simulink model "Controll_RigidBody_R2021b"  (R2021b)
settings: Solver=ode4  StartTime=0.0  StopTime=inf  FixedStep=0.01  MaxStep=0.2  RelTol=1e-3
values from neighbouring files (symbols this model uses):
  Km1 = Km_gain    (= 0.1)    [param_EiH_VFC.m]
  Km2 = Km_gain    (= 0.1)    [param_EiH_VFC.m]
  Km3 = Km_gain    (= 0.1)    [param_EiH_VFC.m]
  Km4 = Km_gain    (= 0.1)    [param_EiH_VFC.m]
  Km5 = Km_gain    (= 0.1)    [param_EiH_VFC.m]
  Km6 = Km_gain    (= 0.1)    [param_EiH_VFC.m]
  R_threshold = 1e-8    (= 1e-08)    [param_EiH_VFC.m]
  zeta_threshold = 1e-8    (= 1e-08)    [param_EiH_VFC.m]
undefined symbols (not defined in the file or in its folder): magnitude, pzeta_d
libraries: dspnetwork x2, dspmtrx3 x1
(part 1 of 2)
settings Model: Creator=toshiyuki  LastModifiedBy=takeh
settings SolverCC: AlgebraicLoopSolver=TrustRegion  InsertRTBMode=Always
settings DataIOCC: ReturnWorkspaceOutputs=off  ReturnWorkspaceOutputsName=tp4a89a2fa_3ce3_4014_a3ba_d599f69fb3ba
settings DebuggingCC: SFMachineParentedDataDiag=warning  ArithmeticOperatorsInVariantConditions=warning
settings SFSimCC: SimUseLocalCustomCode=off  CustomCodeUndefinedFunction=UseInterfaceOnly
settings RTWCC: RTWUseLocalCustomCode=off

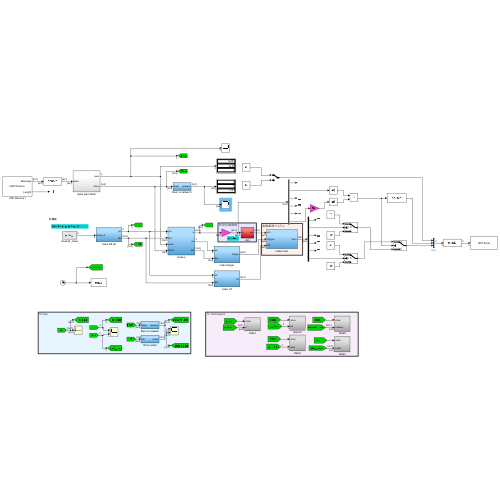
[thumbnail: Simulink's stored preview of the top-level diagram]
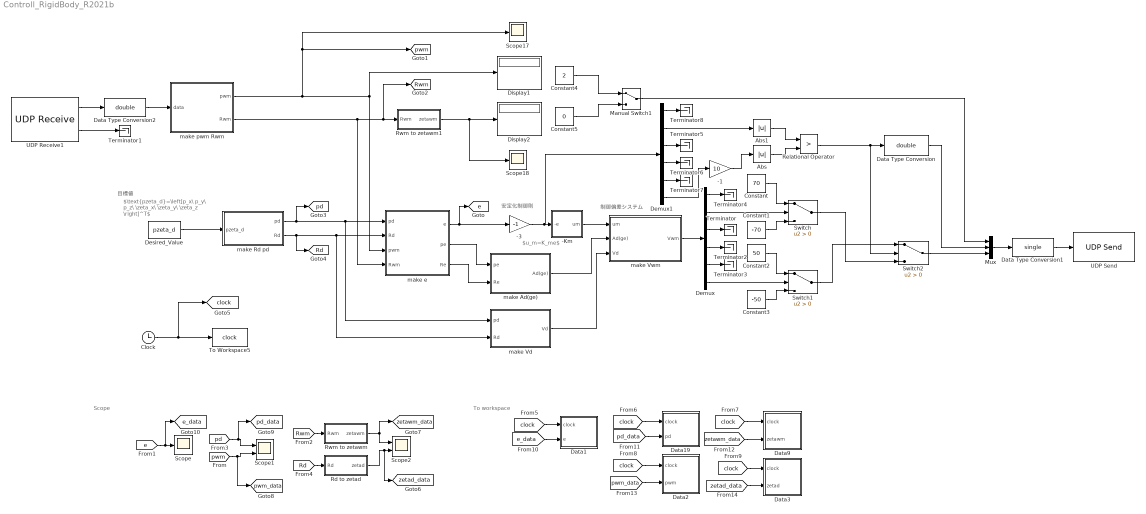
== system Controll_RigidBody_R2021b ==
  note: 制御偏差システム
  note: 目標値
  note: 安定化制御則
  note: $\text{pzeta_d}=\left[p_x\ p_y\ p_z\ \zeta_x\ \zeta_y\ \zeta_z \right]^T$
  note: Scope
  note: To workspace
  note: $u_m=K_me$
  -1 : Gain  Gain=10  SaturateOnIntegerOverflow=on  OutDataTypeStr=Inherit: Same as input  ParamDataTypeStr=Inherit: Same as input
  -3 : Gain  Gain=-1  SaturateOnIntegerOverflow=on  OutDataTypeStr=Inherit: Same as input  ParamDataTypeStr=Inherit: Same as input
  -Km : Subsystem
  Abs : Abs
  Abs1 : Abs
  Clock : Clock
  Constant : Constant  Value=70
  Constant1 : Constant  Value=-70
  Constant2 : Constant  Value=50
  Constant3 : Constant  Value=-50
  Constant4 : Constant  Value=2
  Constant5 : Constant  Value=0
  Data Type Conversion : DataTypeConversion  OutDataTypeStr=double
  Data Type Conversion1 : DataTypeConversion  OutDataTypeStr=single
  Data Type Conversion2 : DataTypeConversion  OutDataTypeStr=double
  Data1 : Subsystem
  Data19 : Subsystem
  Data2 : Subsystem
  Data3 : Subsystem
  Data9 : Subsystem
  Demux : Demux  Outputs=6
  Demux1 : Demux  Outputs=6
  Desired_Value : Constant  Value=pzeta_d
  Display1 : Display
  Display2 : Display
  Manual Switch1 : ManualSwitch
  Mux : Mux  Inputs=3
  Rd to zetad : Subsystem
  Relational Operator : RelationalOperator  Operator=>  OutDataTypeStr=boolean  RndMeth=Simplest
  Rwm to zetawm : Subsystem
  Rwm to zetawm1 : Subsystem
  Scope : Scope
  Scope1 : Scope  NumInputPorts=2
  Scope17 : Scope
  Scope18 : Scope
  Scope2 : Scope  NumInputPorts=2
  Switch : Switch  Criteria=u2 > Threshold
  Switch1 : Switch  Criteria=u2 > Threshold
  Switch2 : Switch  Criteria=u2 > Threshold
  Terminator{,1..8} (9 alike) : Terminator
  To Workspace5 : ToWorkspace  VariableName=clock  SaveFormat=Structure  SampleTime=-1
  UDP Receive1 : dspnetwork/UDP Receive  localURL='0.0.0.0'  localPort=51000  remoteURL='127.0.0.1'  remotePort=-1  recvBufferSize=24  dims=6  signalDatatype=single  isComplex=off  isVarSize=off  showBlockingTime=off  blockingTime=0  sampletime=-1  blockPlatform=[]
  UDP Send : dspnetwork/UDP Send  remoteURL='127.0.0.1'  remotePort=52000  localURL='0.0.0.0'  localPortSource=Automatically determine  localPort=-1  sendBufferSize=8192  sampletime=-1  blockPlatform=[]  separateLengthPort=0
  make Ad(ge) : Subsystem
  make Rd pd : Subsystem
  make Vd : Subsystem
  make Vwm : Subsystem
  make e : Subsystem
  make pwm Rwm : Subsystem
  tag scope: Rd=global, Rwm=global, clock=global, e=global, e_data=global, pd=global, pd_data=global, pwm=global, pwm_data=global, zetad_data=global, zetawm_data=global
  wires:
  make Rd pd/1(pd) -> [pd], make e/1(pd), make Vd/1(pd)
  make Rd pd/2(Rd) -> [Rd], make e/2(Rd), make Vd/2(Rd)
  Desired_Value/1 -> make Rd pd/1(pzeta_d)
  make e/1(e) -> [e], -3/1
  make e/2(pe) -> make Ad(ge)/1(pe)
  make e/3(Re) -> make Ad(ge)/2(Re)
  -Km/1(um) -> make Vwm/1(um)
  make Ad(ge)/1(Ad(ge)) -> make Vwm/2(Ad(ge))
  make Vd/1(Vd) -> make Vwm/3(Vd)
  make Vwm/1(Vwm) -> Demux/1
  make pwm Rwm/2(Rwm) -> [Rwm], Rwm to zetawm1/1(Rwm), make e/4(Rwm)
  make pwm Rwm/1(pwm) -> [pwm], Scope17/1, make e/3(pwm), Display1/1
  [e] -> [e_data], Scope/1
  [pd] -> [pd_data], Scope1/1
  [pwm] -> [pwm_data], Scope1/2
  [Rwm] -> Rwm to zetawm/1(Rwm)
  [Rd] -> Rd to zetad/1(Rd)
  Rwm to zetawm/1(zetawm) -> [zetawm_data], Scope2/1
  Rd to zetad/1(zetad) -> [zetad_data], Scope2/2
  Clock/1 -> [clock], To Workspace5/1
  [clock] -> Data1/1(clock)
  [clock] -> Data19/1(clock)
  [clock] -> Data9/1(clock)
  [clock] -> Data2/1(clock)
  [clock] -> Data3/1(clock)
  [zetawm_data] -> Data9/2(zetawm)
  [zetad_data] -> Data3/2(zetad)
  [pd_data] -> Data19/2(pd)
  [pwm_data] -> Data2/2(pwm)
  [e_data] -> Data1/2(e)
  UDP Receive1/1 -> Data Type Conversion2/1
  UDP Receive1/2 -> Terminator1/1
  Data Type Conversion2/1 -> make pwm Rwm/1(data)
  Rwm to zetawm1/1(zetawm) -> Scope18/1, Display2/1
  Demux/3 -> Terminator/1
  Demux/4 -> Terminator2/1
  Demux/5 -> Terminator3/1
  Demux/1 -> Terminator4/1
  Demux/2 -> Switch/2
  Constant/1 -> Switch/1
  Constant1/1 -> Switch/3
  Demux/6 -> Switch1/2
  Constant2/1 -> Switch1/1
  Constant3/1 -> Switch1/3
  Data Type Conversion1/1 -> UDP Send/1
  Mux/1 -> Data Type Conversion1/1
  Constant4/1 -> Manual Switch1/1
  Constant5/1 -> Manual Switch1/2
  Demux1/4 -> Terminator6/1
  Demux1/5 -> Terminator7/1
  Demux1/1 -> Terminator8/1
  Demux1/2 -> Abs1/1
  Demux1/3 -> Terminator5/1
  Demux1/6 -> -1/1
  -3/1 -> Demux1/1, -Km/1(-e)
  -1/1 -> Abs/1
  Abs1/1 -> Relational Operator/1
  Abs/1 -> Relational Operator/2
  Relational Operator/1 -> Switch2/2, Data Type Conversion/1
  Manual Switch1/1 -> Mux/1
  Switch/1 -> Switch2/3
  Switch2/1 -> Mux/3
  Switch1/1 -> Switch2/1
  Data Type Conversion/1 -> Mux/2

== system Controll_RigidBody_R2021b/-Km ==
  -e : Inport
  Gain : Gain  Gain=-1  Multiplication=Matrix(K*u)  SaturateOnIntegerOverflow=on  OutDataTypeStr=Inherit: Same as input  ParamDataTypeStr=Inherit: Same as input
  Kcc : Subsystem
  Product : Product  Multiplication=Matrix(*)  InputSameDT=on  SaturateOnIntegerOverflow=on  OutDataTypeStr=Inherit: Same as first input
  um : Outport  VectorParamsAs1DForOutWhenUnconnected=off
  wires:
  Gain/1 -> Product/1
  Kcc/1(Km) -> Gain/1
  Product/1 -> um/1
  -e/1 -> Product/2

== system Controll_RigidBody_R2021b/Data1 ==
  clock : Inport
  e : Inport  Port=2
  Demux4 : Demux  Outputs=6
      settings: DisplayOption=none
  Mux2 : Mux  Inputs=7
  To Workspace1 : ToWorkspace  VariableName=e  SaveFormat=Structure  SampleTime=-1
  wires:
  Demux4/6 -> Mux2/7
  Demux4/5 -> Mux2/6
  Demux4/4 -> Mux2/5
  Demux4/3 -> Mux2/4
  Demux4/2 -> Mux2/3
  Demux4/1 -> Mux2/2
  clock/1 -> Mux2/1
  Mux2/1 -> To Workspace1/1
  e/1 -> Demux4/1

== system Controll_RigidBody_R2021b/Data19 ==
  clock : Inport
  pd : Inport  Port=2
  Demux4 : Demux  Outputs=3
      settings: DisplayOption=none
  Mux2 : Mux
  To Workspace1 : ToWorkspace  VariableName=pd  SaveFormat=Structure  SampleTime=-1
  wires:
  pd/1 -> Demux4/1
  clock/1 -> Mux2/1
  Mux2/1 -> To Workspace1/1
  Demux4/3 -> Mux2/4
  Demux4/2 -> Mux2/3
  Demux4/1 -> Mux2/2

== system Controll_RigidBody_R2021b/Data2 ==
  clock : Inport
  pwm : Inport  Port=2
  Demux4 : Demux  Outputs=3
      settings: DisplayOption=none
  Mux2 : Mux
  To Workspace1 : ToWorkspace  VariableName=pwm  SaveFormat=Structure  SampleTime=-1
  wires:
  Demux4/1 -> Mux2/2
  Demux4/2 -> Mux2/3
  Demux4/3 -> Mux2/4
  Mux2/1 -> To Workspace1/1
  clock/1 -> Mux2/1
  pwm/1 -> Demux4/1

== system Controll_RigidBody_R2021b/Data3 ==
  clock : Inport
  zetad : Inport  Port=2
  Demux4 : Demux  Outputs=3
      settings: DisplayOption=none
  Mux2 : Mux
  To Workspace1 : ToWorkspace  VariableName=zetad  SaveFormat=Structure  SampleTime=-1
  wires:
  zetad/1 -> Demux4/1
  clock/1 -> Mux2/1
  Mux2/1 -> To Workspace1/1
  Demux4/3 -> Mux2/4
  Demux4/2 -> Mux2/3
  Demux4/1 -> Mux2/2

== system Controll_RigidBody_R2021b/Data9 ==
  clock : Inport
  zetawm : Inport  Port=2
  Demux4 : Demux  Outputs=3
      settings: DisplayOption=none
  Mux2 : Mux
  To Workspace1 : ToWorkspace  VariableName=zetawm  SaveFormat=Structure  SampleTime=-1
  wires:
  Demux4/1 -> Mux2/2
  Demux4/2 -> Mux2/3
  Demux4/3 -> Mux2/4
  Mux2/1 -> To Workspace1/1
  clock/1 -> Mux2/1
  zetawm/1 -> Demux4/1

== system Controll_RigidBody_R2021b/Rd to zetad ==
  Rd : Inport
  e_R(R) : Subsystem
  make zeta : Subsystem
  zetad : Outport  VectorParamsAs1DForOutWhenUnconnected=off
  wires:
  make zeta/1(zeta) -> zetad/1
  Rd/1 -> e_R(R)/1(R)
  e_R(R)/1(sk(R)^vee) -> make zeta/1(sk(R)^vee)

== system Controll_RigidBody_R2021b/Rwm to zetawm ==
  Rwm : Inport
  e_R(R) : Subsystem
  make zeta : Subsystem
  zetawm : Outport  VectorParamsAs1DForOutWhenUnconnected=off
  wires:
  make zeta/1(zeta) -> zetawm/1
  Rwm/1 -> e_R(R)/1(R)
  e_R(R)/1(sk(R)^vee) -> make zeta/1(sk(R)^vee)

== system Controll_RigidBody_R2021b/Rwm to zetawm1 ==
  Rwm : Inport
  e_R(R) : Subsystem
  make zeta : Subsystem
  zetawm : Outport  VectorParamsAs1DForOutWhenUnconnected=off
  wires:
  make zeta/1(zeta) -> zetawm/1
  Rwm/1 -> e_R(R)/1(R)
  e_R(R)/1(sk(R)^vee) -> make zeta/1(sk(R)^vee)

== system Controll_RigidBody_R2021b/make Ad(ge) ==
  note: $\hat{p_e}R_e$
  note: $\left(R_e\ \hat{p_e}R_e\right)$
  note: $\left(0\ R_e\right)$
  note: $\text{Ad}_{(g_e)}=\left[\begin{array}{cc} R_e & \hat{p_e}R_e\\ 0&R_e \end{array}\right]$
  pe : Inport
  Re : Inport  Port=2
  Gain : Gain  Gain=0  Multiplication=Matrix(K*u)
  Identity Matrix : dspmtrx3/Identity Matrix  Inherit=off  N=3  Ts=1  dataType=double  isSigned=on  wordLen=16  udDataType=sfix(16)  fracBitsMode=Best precision  numFracBits=15  OutDataTypeStr=double  LastOutDataTypeStr=double
  Matrix Concatenate : Concatenate  Mode=Multidimensional array  ConcatenateDimension=2
  Matrix Concatenate1 : Concatenate  Mode=Multidimensional array  ConcatenateDimension=2
  Matrix Concatenate2 : Concatenate  Mode=Multidimensional array
  Product2 : Product  Multiplication=Matrix(*)
  wedge : Subsystem
  Ad(ge) : Outport  VectorParamsAs1DForOutWhenUnconnected=off
  wires:
  pe/1 -> wedge/1("[3x1]")
  wedge/1("[3x3]") -> Product2/1
  Re/1 -> Matrix Concatenate1/2, Product2/2, Matrix Concatenate/1
  Product2/1 -> Matrix Concatenate/2
  Matrix Concatenate/1 -> Matrix Concatenate2/1
  Matrix Concatenate1/1 -> Matrix Concatenate2/2
  Matrix Concatenate2/1 -> Ad(ge)/1
  Identity Matrix/1 -> Gain/1
  Gain/1 -> Matrix Concatenate1/1

== system Controll_RigidBody_R2021b/make Rd pd ==
  note: 目標姿勢
  note: 目標位置
  note: $p_d=\left(p_x \ p_y\ p_z\right)^T$$
  note: $\zeta_d=\left(\zeta_x \ \zeta_y\ \zeta_z\right)^T\text{\ \ →\ \ 回転行列}R_d$
  pzeta_d : Inport
  Demux3 : Demux  Outputs=6
      settings: DisplayOption=none
  Mux : Mux  Inputs=3
  Mux1 : Mux  Inputs=3
  make_Rd : Subsystem
  pd : Outport  VectorParamsAs1DForOutWhenUnconnected=off
  Rd : Outport  Port=2  VectorParamsAs1DForOutWhenUnconnected=off
  wires:
  Demux3/2 -> Mux1/2
  Demux3/1 -> Mux1/1
  Demux3/5 -> Mux/2
  Demux3/4 -> Mux/1
  pzeta_d/1 -> Demux3/1
  Mux/1 -> make_Rd/1(zeta_d)
  Demux3/3 -> Mux1/3
  Demux3/6 -> Mux/3
  Mux1/1 -> pd/1
  make_Rd/1(Rd) -> Rd/1

== system Controll_RigidBody_R2021b/make Vd ==
  note: $v_d^b=R_{d}^T\dot{p}_{d}$
  note: $\omega_d^b=\left(R_{d}^T\dot{R}_{d}\right)^\vee$
  note: $V_d^b=\left[\begin{array}{c} v_d^b\\ \omega_d^b \end{array} \right]$
  pd : Inport
  Rd : Inport  Port=2
  Derivative : Derivative
  Derivative1 : Derivative
  Math Function : Math  Operator=transpose  SignedPower=on  SaturateOnIntegerOverflow=on
  Mux : Mux  Inputs=2
  Product1 : Product  Multiplication=Matrix(*)
  Product2 : Product  Multiplication=Matrix(*)
  vee : Subsystem
  Vd : Outport  VectorParamsAs1DForOutWhenUnconnected=off
  wires:
  pd/1 -> Derivative/1
  Rd/1 -> Derivative1/1, Math Function/1
  Math Function/1 -> Product2/1, Product1/1
  Derivative1/1 -> Product1/2
  Product1/1 -> vee/1("[3*3]")
  vee/1("[3*1]") -> Mux/2
  Product2/1 -> Mux/1
  Mux/1 -> Vd/1
  Derivative/1 -> Product2/2

== system Controll_RigidBody_R2021b/make Vwm ==
  note: $\text{Ad}_{(g_e)}\ \ \text{→}\ \ \text{Ad}_{(g_e)}^{-1}$
  note: $V_{wm}=-\text{Ad}_{(g_e)}^{-1}\left(u_m-V_d\right)$
  um : Inport
  Ad(ge) : Inport  Port=2
  Vd : Inport  Port=3
  -3 : Gain  Gain=-1  SaturateOnIntegerOverflow=on  OutDataTypeStr=Inherit: Same as input  ParamDataTypeStr=Inherit: Same as input
  MATLAB Function : MATLAB Function  TreatAsAtomicUnit=on
  Product2 : Product  Multiplication=Matrix(*)
  Sum : Sum  Inputs=|+-
  Vwm : Outport  VectorParamsAs1DForOutWhenUnconnected=off
  wires:
  Product2/1 -> Vwm/1
  Ad(ge)/1 -> MATLAB Function/1(Ad_ge)
  um/1 -> Sum/1
  Vd/1 -> Sum/2
  MATLAB Function/1(inv_Ad_ge) -> -3/1
  -3/1 -> Product2/1
  Sum/1 -> Product2/2

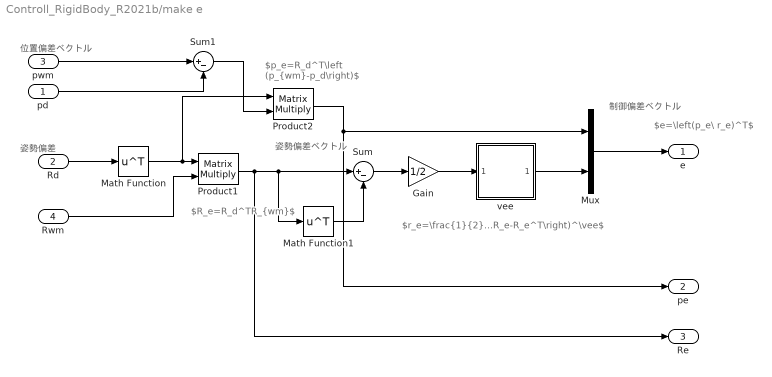
== system Controll_RigidBody_R2021b/make e ==
  note: 制御偏差ベクトル
  note: 姿勢偏差ベクトル
  note: 姿勢偏差
  note: 位置偏差ベクトル
  note: $p_e=R_d^T\left (p_{wm}-p_d\right)$
  note: $R_e=R_d^TR_{wm}$
  note: $r_e=\frac{1}{2}\left(R_e-R_e^T\right)^\vee$
  note: $e=\left(p_e\ r_e)^T$
  pd : Inport
  Rd : Inport  Port=2
  pwm : Inport  Port=3
  Rwm : Inport  Port=4
  Gain : Gain  Gain=1/2
  Math Function : Math  Operator=transpose  SignedPower=on  SaturateOnIntegerOverflow=on
  Math Function1 : Math  Operator=transpose  SignedPower=on  SaturateOnIntegerOverflow=on
  Mux : Mux  Inputs=2
  Product1 : Product  Multiplication=Matrix(*)
  Product2 : Product  Multiplication=Matrix(*)
  Sum : Sum  Inputs=|+-
  Sum1 : Sum  Inputs=|+-
  vee : Subsystem
  e : Outport  VectorParamsAs1DForOutWhenUnconnected=off
  pe : Outport  Port=2  VectorParamsAs1DForOutWhenUnconnected=off
  Re : Outport  Port=3  VectorParamsAs1DForOutWhenUnconnected=off
  wires:
  Rd/1 -> Math Function/1
  Math Function/1 -> Product2/1, Product1/1
  Rwm/1 -> Product1/2
  pwm/1 -> Sum1/1
  pd/1 -> Sum1/2
  Sum1/1 -> Product2/2
  vee/1("[3*1]") -> Mux/2
  Sum/1 -> Gain/1
  Math Function1/1 -> Sum/2
  Product2/1 -> pe/1, Mux/1
  Gain/1 -> vee/1("[3*3]")
  Mux/1 -> e/1
  Product1/1 -> Re/1, Math Function1/1, Sum/1

== system Controll_RigidBody_R2021b/make pwm Rwm ==
  data : Inport
  Constant : Constant  Value=0
  Demux : Demux  Outputs=6
  Mux1 : Mux  Inputs=3
  Mux2 : Mux  Inputs=3
  Sum5 : Sum  Inputs=|+-
  Sum6 : Sum  Inputs=|+-
  Sum7 : Sum  Inputs=+-|
  make_Rd : Subsystem
  pwm : Outport
  Rwm : Outport  Port=2
  wires:
  Sum6/1 -> Mux1/2
  Demux/6 -> Sum7/2
  Demux/4 -> Sum5/2
  Sum5/1 -> Mux1/1
  Demux/3 -> Sum7/1
  Demux/2 -> Sum6/1
  Demux/1 -> Sum5/1
  Demux/5 -> Sum6/2
  data/1 -> Demux/1
  Constant/1 -> Mux2/2, Mux2/1, Mux1/3
  Mux1/1 -> pwm/1
  Sum7/1 -> Mux2/3
  Mux2/1 -> make_Rd/1(zeta_d)
  make_Rd/1(Rd) -> Rwm/1

== system Controll_RigidBody_R2021b/-Km/Kcc ==
  Ke1 : Constant  Value=Km1
  Ke2 : Constant  Value=Km2
  Ke3 : Constant  Value=Km3
  Ke4 : Constant  Value=Km4
  Ke5 : Constant  Value=Km5
  Ke6 : Constant  Value=Km6
  Mux : Mux  Inputs=6
  diag : Subsystem
  Km : Outport  VectorParamsAs1DForOutWhenUnconnected=off
  wires:
  Mux/1 -> diag/1(in[6*1])
  Ke6/1 -> Mux/6
  Ke5/1 -> Mux/5
  Ke4/1 -> Mux/4
  Ke3/1 -> Mux/3
  Ke2/1 -> Mux/2
  Ke1/1 -> Mux/1
  diag/1(diag) -> Km/1

== system Controll_RigidBody_R2021b/Rd to zetad/e_R(R) ==
  R : Inport
  sk(R) : Subsystem
  vee : Subsystem
  sk(R)^vee : Outport  VectorParamsAs1DForOutWhenUnconnected=off
  wires:
  R/1 -> sk(R)/1(R)
  vee/1("[3*1]") -> sk(R)^vee/1
  sk(R)/1(sk(R)) -> vee/1("[3*3]")

== system Controll_RigidBody_R2021b/Rd to zetad/make zeta ==
  sk(R)^vee : Inport
  "3x1 -> 2norm" : Subsystem
  Product : Product  InputSameDT=on  SaturateOnIntegerOverflow=on  OutDataTypeStr=Inherit: Same as first input
  Product1 : Product  Inputs=/  InputSameDT=on  SaturateOnIntegerOverflow=on  OutDataTypeStr=Inherit: Same as first input
  Product2 : Product  InputSameDT=on  SaturateOnIntegerOverflow=on  OutDataTypeStr=Inherit: Same as first input
  Switch : Switch  Threshold=zeta_threshold  SaturateOnIntegerOverflow=on  InputSameDT=on
  Trigonometric Function : Trigonometry  Operator=asin
  zero : Constant  Value=[0;0;0]  VectorParams1D=off
  zero check zeta_threshold : Subsystem
  zeta : Outport  VectorParamsAs1DForOutWhenUnconnected=off
  wires:
  zero/1 -> Switch/3
  Product/1 -> Switch/1
  Switch/1 -> zeta/1
  zero check zeta_threshold/1(Out1) -> Switch/2, Product1/1, Trigonometric Function/1
  sk(R)^vee/1 -> "3x1 -> 2norm"/1(3x1), Product/2
  "3x1 -> 2norm"/1(2 norm) -> zero check zeta_threshold/1(In1)
  Trigonometric Function/1 -> Product2/1
  Product1/1 -> Product2/2
  Product2/1 -> Product/1

== system Controll_RigidBody_R2021b/Rwm to zetawm/e_R(R) ==
  R : Inport
  sk(R) : Subsystem
  vee : Subsystem
  sk(R)^vee : Outport  VectorParamsAs1DForOutWhenUnconnected=off
  wires:
  R/1 -> sk(R)/1(R)
  vee/1("[3*1]") -> sk(R)^vee/1
  sk(R)/1(sk(R)) -> vee/1("[3*3]")

== system Controll_RigidBody_R2021b/Rwm to zetawm/make zeta ==
  sk(R)^vee : Inport
  "3x1 -> 2norm" : Subsystem
  Product : Product  InputSameDT=on  SaturateOnIntegerOverflow=on  OutDataTypeStr=Inherit: Same as first input
  Product1 : Product  Inputs=/  InputSameDT=on  SaturateOnIntegerOverflow=on  OutDataTypeStr=Inherit: Same as first input
  Product2 : Product  InputSameDT=on  SaturateOnIntegerOverflow=on  OutDataTypeStr=Inherit: Same as first input
  Switch : Switch  Threshold=zeta_threshold  SaturateOnIntegerOverflow=on  InputSameDT=on
  Trigonometric Function : Trigonometry  Operator=asin
  zero : Constant  Value=[0;0;0]  VectorParams1D=off
  zero check zeta_threshold : Subsystem
  zeta : Outport  VectorParamsAs1DForOutWhenUnconnected=off
  wires:
  zero/1 -> Switch/3
  Product/1 -> Switch/1
  Switch/1 -> zeta/1
  zero check zeta_threshold/1(Out1) -> Switch/2, Product1/1, Trigonometric Function/1
  sk(R)^vee/1 -> "3x1 -> 2norm"/1(3x1), Product/2
  "3x1 -> 2norm"/1(2 norm) -> zero check zeta_threshold/1(In1)
  Trigonometric Function/1 -> Product2/1
  Product1/1 -> Product2/2
  Product2/1 -> Product/1

== system Controll_RigidBody_R2021b/Rwm to zetawm1/e_R(R) ==
  R : Inport
  sk(R) : Subsystem
  vee : Subsystem
  sk(R)^vee : Outport  VectorParamsAs1DForOutWhenUnconnected=off
  wires:
  R/1 -> sk(R)/1(R)
  vee/1("[3*1]") -> sk(R)^vee/1
  sk(R)/1(sk(R)) -> vee/1("[3*3]")

== system Controll_RigidBody_R2021b/Rwm to zetawm1/make zeta ==
  sk(R)^vee : Inport
  "3x1 -> 2norm" : Subsystem
  Product : Product  InputSameDT=on  SaturateOnIntegerOverflow=on  OutDataTypeStr=Inherit: Same as first input
  Product1 : Product  Inputs=/  InputSameDT=on  SaturateOnIntegerOverflow=on  OutDataTypeStr=Inherit: Same as first input
  Product2 : Product  InputSameDT=on  SaturateOnIntegerOverflow=on  OutDataTypeStr=Inherit: Same as first input
  Switch : Switch  Threshold=zeta_threshold  SaturateOnIntegerOverflow=on  InputSameDT=on
  Trigonometric Function : Trigonometry  Operator=asin
  zero : Constant  Value=[0;0;0]  VectorParams1D=off
  zero check zeta_threshold : Subsystem
  zeta : Outport  VectorParamsAs1DForOutWhenUnconnected=off
  wires:
  zero/1 -> Switch/3
  Product/1 -> Switch/1
  Switch/1 -> zeta/1
  zero check zeta_threshold/1(Out1) -> Switch/2, Product1/1, Trigonometric Function/1
  sk(R)^vee/1 -> "3x1 -> 2norm"/1(3x1), Product/2
  "3x1 -> 2norm"/1(2 norm) -> zero check zeta_threshold/1(In1)
  Trigonometric Function/1 -> Product2/1
  Product1/1 -> Product2/2
  Product2/1 -> Product/1

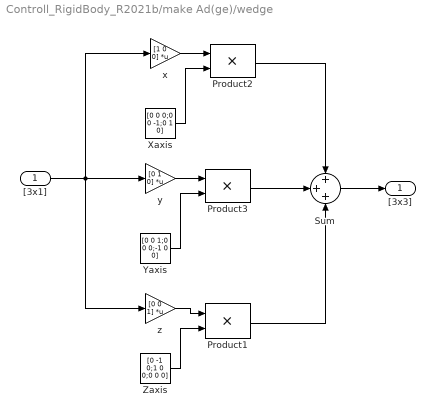
== system Controll_RigidBody_R2021b/make Ad(ge)/wedge ==
  "[3x1]" : Inport
  Product1 : Product  InputSameDT=on  SaturateOnIntegerOverflow=on  OutDataTypeStr=Inherit: Same as first input
  Product2 : Product  InputSameDT=on  SaturateOnIntegerOverflow=on  OutDataTypeStr=Inherit: Same as first input
  Product3 : Product  InputSameDT=on  SaturateOnIntegerOverflow=on  OutDataTypeStr=Inherit: Same as first input
  Sum : Sum  Inputs=+++  InputSameDT=on  SaturateOnIntegerOverflow=on  OutDataTypeStr=Inherit: Same as first input
  Xaxis : Constant  Value=[0 0 0;0 0 -1;0 1 0]  VectorParams1D=off
  Yaxis : Constant  Value=[0 0 1;0 0 0;-1 0 0]  VectorParams1D=off
  Zaxis : Constant  Value=[0 -1 0;1 0 0;0 0 0]  VectorParams1D=off
  x : Gain  Gain=[1 0 0]  Multiplication=Matrix(K*u)  SaturateOnIntegerOverflow=on  OutDataTypeStr=Inherit: Same as input  ParamDataTypeStr=Inherit: Same as input
  y : Gain  Gain=[0 1 0]  Multiplication=Matrix(K*u)  SaturateOnIntegerOverflow=on  OutDataTypeStr=Inherit: Same as input  ParamDataTypeStr=Inherit: Same as input
  z : Gain  Gain=[0 0 1]  Multiplication=Matrix(K*u)  SaturateOnIntegerOverflow=on  OutDataTypeStr=Inherit: Same as input  ParamDataTypeStr=Inherit: Same as input
  "[3x3]" : Outport  VectorParamsAs1DForOutWhenUnconnected=off
  wires:
  Sum/1 -> "[3x3]"/1
  Product1/1 -> Sum/3
  Product2/1 -> Sum/1
  Product3/1 -> Sum/2
  "[3x1]"/1 -> z/1, x/1, y/1
  y/1 -> Product3/1
  Yaxis/1 -> Product3/2
  x/1 -> Product2/1
  Xaxis/1 -> Product2/2
  z/1 -> Product1/1
  Zaxis/1 -> Product1/2

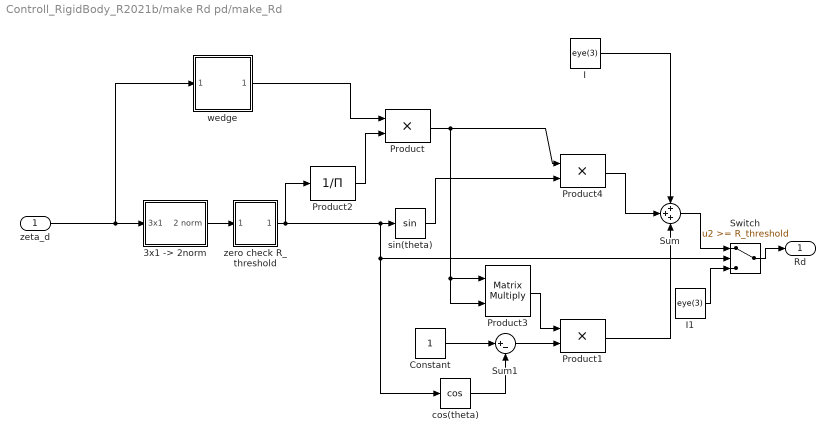
== system Controll_RigidBody_R2021b/make Rd pd/make_Rd ==
  zeta_d : Inport
  "3x1 -> 2norm" : Subsystem
  Constant : Constant
  I : Constant  Value=eye(3)  VectorParams1D=off
  I1 : Constant  Value=eye(3)  VectorParams1D=off
  Product : Product  InputSameDT=on  SaturateOnIntegerOverflow=on  OutDataTypeStr=Inherit: Same as first input
  Product1 : Product  InputSameDT=on  SaturateOnIntegerOverflow=on  OutDataTypeStr=Inherit: Same as first input
  Product2 : Product  Inputs=/  InputSameDT=on  SaturateOnIntegerOverflow=on  OutDataTypeStr=Inherit: Same as first input
  Product3 : Product  Multiplication=Matrix(*)  InputSameDT=on  SaturateOnIntegerOverflow=on  OutDataTypeStr=Inherit: Same as first input
  Product4 : Product  InputSameDT=on  SaturateOnIntegerOverflow=on  OutDataTypeStr=Inherit: Same as first input
  Sum : Sum  Inputs=+++  InputSameDT=on  SaturateOnIntegerOverflow=on  OutDataTypeStr=Inherit: Same as first input
  Sum1 : Sum  Inputs=|+-  InputSameDT=on  SaturateOnIntegerOverflow=on  OutDataTypeStr=Inherit: Same as first input
  Switch : Switch  Threshold=R_threshold  SaturateOnIntegerOverflow=on  InputSameDT=on
  cos(theta) : Trigonometry  Operator=cos
  sin(theta) : Trigonometry
  wedge : Subsystem
  zero check R_threshold : Subsystem
  Rd : Outport  VectorParamsAs1DForOutWhenUnconnected=off
  wires:
  Product3/1 -> Product1/1
  zeta_d/1 -> wedge/1("[3x1]"), "3x1 -> 2norm"/1(3x1)
  Product2/1 -> Product/2
  zero check R_threshold/1(Out1) -> cos(theta)/1, Switch/2, sin(theta)/1, Product2/1
  wedge/1("[3x3]") -> Product/1
  Product/1 -> Product3/2, Product3/1, Product4/1
  "3x1 -> 2norm"/1(2 norm) -> zero check R_threshold/1(In1)
  Switch/1 -> Rd/1
  I1/1 -> Switch/3
  Sum/1 -> Switch/1
  sin(theta)/1 -> Product4/2
  I/1 -> Sum/1
  Constant/1 -> Sum1/1
  cos(theta)/1 -> Sum1/2
  Sum1/1 -> Product1/2
  Product1/1 -> Sum/3
  Product4/1 -> Sum/2

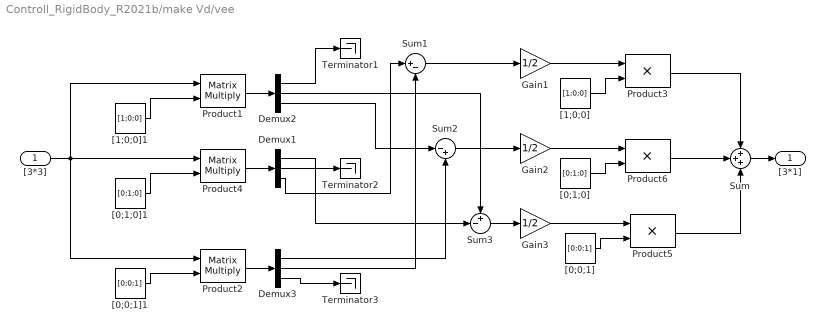
== system Controll_RigidBody_R2021b/make Vd/vee ==
  "[3*3]" : Inport
  Demux1 : Demux  Outputs=3
      settings: DisplayOption=none
  Demux2 : Demux  Outputs=3
      settings: DisplayOption=none
  Demux3 : Demux  Outputs=3
      settings: DisplayOption=none
  Gain1 : Gain  Gain=1/2  SaturateOnIntegerOverflow=on  OutDataTypeStr=Inherit: Same as input  ParamDataTypeStr=Inherit: Same as input
  Gain2 : Gain  Gain=1/2  SaturateOnIntegerOverflow=on  OutDataTypeStr=Inherit: Same as input  ParamDataTypeStr=Inherit: Same as input
  Gain3 : Gain  Gain=1/2  SaturateOnIntegerOverflow=on  OutDataTypeStr=Inherit: Same as input  ParamDataTypeStr=Inherit: Same as input
  Product1 : Product  Multiplication=Matrix(*)  InputSameDT=on  SaturateOnIntegerOverflow=on  OutDataTypeStr=Inherit: Same as first input
  Product2 : Product  Multiplication=Matrix(*)  InputSameDT=on  SaturateOnIntegerOverflow=on  OutDataTypeStr=Inherit: Same as first input
  Product3 : Product  InputSameDT=on  SaturateOnIntegerOverflow=on  OutDataTypeStr=Inherit: Same as first input
  Product4 : Product  Multiplication=Matrix(*)  InputSameDT=on  SaturateOnIntegerOverflow=on  OutDataTypeStr=Inherit: Same as first input
  Product5 : Product  InputSameDT=on  SaturateOnIntegerOverflow=on  OutDataTypeStr=Inherit: Same as first input
  Product6 : Product  InputSameDT=on  SaturateOnIntegerOverflow=on  OutDataTypeStr=Inherit: Same as first input
  Sum : Sum  Inputs=+++  InputSameDT=on  SaturateOnIntegerOverflow=on  OutDataTypeStr=Inherit: Same as first input
  Sum1 : Sum  Inputs=|+-  InputSameDT=on  SaturateOnIntegerOverflow=on  OutDataTypeStr=Inherit: Same as first input
  Sum2 : Sum  Inputs=|-+  InputSameDT=on  SaturateOnIntegerOverflow=on  OutDataTypeStr=Inherit: Same as first input
  Sum3 : Sum  Inputs=+-|  InputSameDT=on  SaturateOnIntegerOverflow=on  OutDataTypeStr=Inherit: Same as first input
  Terminator1 : Terminator
  Terminator2 : Terminator
  Terminator3 : Terminator
  "[0;0;1]" : Constant  Value=[0;0;1]  VectorParams1D=off
  "[0;0;1]1" : Constant  Value=[0;0;1]  VectorParams1D=off
  "[0;1;0]" : Constant  Value=[0;1;0]  VectorParams1D=off
  "[0;1;0]1" : Constant  Value=[0;1;0]  VectorParams1D=off
  "[1;0;0]" : Constant  Value=[1;0;0]  VectorParams1D=off
  "[1;0;0]1" : Constant  Value=[1;0;0]  VectorParams1D=off
  "[3*1]" : Outport  VectorParamsAs1DForOutWhenUnconnected=off
  wires:
  Demux1/1 -> Sum3/2
  Demux2/2 -> Sum3/1
  Sum3/1 -> Gain3/1
  Sum2/1 -> Gain2/1
  Demux2/3 -> Sum2/1
  Gain3/1 -> Product5/1
  Gain2/1 -> Product6/1
  Demux3/2 -> Sum1/2
  Gain1/1 -> Product3/1
  Sum1/1 -> Gain1/1
  Sum/1 -> "[3*1]"/1
  Product3/1 -> Sum/1
  Product5/1 -> Sum/3
  Product6/1 -> Sum/2
  "[0;0;1]"/1 -> Product5/2
  "[0;1;0]"/1 -> Product6/2
  "[1;0;0]"/1 -> Product3/2
  Demux3/1 -> Sum2/2
  Demux3/3 -> Terminator3/1
  Product2/1 -> Demux3/1
  "[0;0;1]1"/1 -> Product2/2
  Demux2/1 -> Terminator1/1
  Product1/1 -> Demux2/1
  "[1;0;0]1"/1 -> Product1/2
  Demux1/3 -> Sum1/1
  Demux1/2 -> Terminator2/1
  Product4/1 -> Demux1/1
  "[0;1;0]1"/1 -> Product4/2
  "[3*3]"/1 -> Product1/1, Product2/1, Product4/1

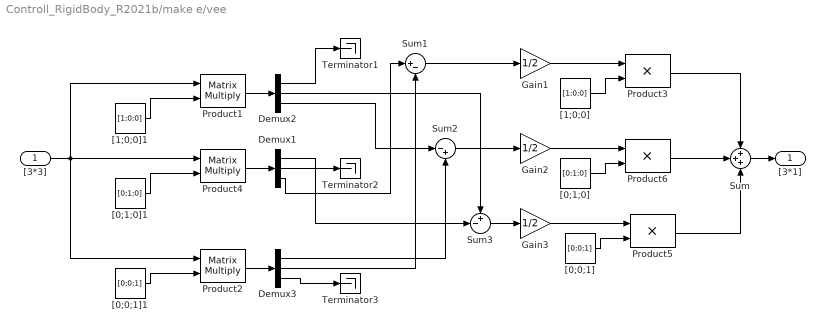
== system Controll_RigidBody_R2021b/make e/vee ==
  "[3*3]" : Inport
  Demux1 : Demux  Outputs=3
      settings: DisplayOption=none
  Demux2 : Demux  Outputs=3
      settings: DisplayOption=none
  Demux3 : Demux  Outputs=3
      settings: DisplayOption=none
  Gain1 : Gain  Gain=1/2  SaturateOnIntegerOverflow=on  OutDataTypeStr=Inherit: Same as input  ParamDataTypeStr=Inherit: Same as input
  Gain2 : Gain  Gain=1/2  SaturateOnIntegerOverflow=on  OutDataTypeStr=Inherit: Same as input  ParamDataTypeStr=Inherit: Same as input
  Gain3 : Gain  Gain=1/2  SaturateOnIntegerOverflow=on  OutDataTypeStr=Inherit: Same as input  ParamDataTypeStr=Inherit: Same as input
  Product1 : Product  Multiplication=Matrix(*)  InputSameDT=on  SaturateOnIntegerOverflow=on  OutDataTypeStr=Inherit: Same as first input
  Product2 : Product  Multiplication=Matrix(*)  InputSameDT=on  SaturateOnIntegerOverflow=on  OutDataTypeStr=Inherit: Same as first input
  Product3 : Product  InputSameDT=on  SaturateOnIntegerOverflow=on  OutDataTypeStr=Inherit: Same as first input
  Product4 : Product  Multiplication=Matrix(*)  InputSameDT=on  SaturateOnIntegerOverflow=on  OutDataTypeStr=Inherit: Same as first input
  Product5 : Product  InputSameDT=on  SaturateOnIntegerOverflow=on  OutDataTypeStr=Inherit: Same as first input
  Product6 : Product  InputSameDT=on  SaturateOnIntegerOverflow=on  OutDataTypeStr=Inherit: Same as first input
  Sum : Sum  Inputs=+++  InputSameDT=on  SaturateOnIntegerOverflow=on  OutDataTypeStr=Inherit: Same as first input
  Sum1 : Sum  Inputs=|+-  InputSameDT=on  SaturateOnIntegerOverflow=on  OutDataTypeStr=Inherit: Same as first input
  Sum2 : Sum  Inputs=|-+  InputSameDT=on  SaturateOnIntegerOverflow=on  OutDataTypeStr=Inherit: Same as first input
  Sum3 : Sum  Inputs=+-|  InputSameDT=on  SaturateOnIntegerOverflow=on  OutDataTypeStr=Inherit: Same as first input
  Terminator1 : Terminator
  Terminator2 : Terminator
  Terminator3 : Terminator
  "[0;0;1]" : Constant  Value=[0;0;1]  VectorParams1D=off
  "[0;0;1]1" : Constant  Value=[0;0;1]  VectorParams1D=off
  "[0;1;0]" : Constant  Value=[0;1;0]  VectorParams1D=off
  "[0;1;0]1" : Constant  Value=[0;1;0]  VectorParams1D=off
  "[1;0;0]" : Constant  Value=[1;0;0]  VectorParams1D=off
  "[1;0;0]1" : Constant  Value=[1;0;0]  VectorParams1D=off
  "[3*1]" : Outport  VectorParamsAs1DForOutWhenUnconnected=off
  wires:
  Demux1/1 -> Sum3/2
  Demux2/2 -> Sum3/1
  Sum3/1 -> Gain3/1
  Sum2/1 -> Gain2/1
  Demux2/3 -> Sum2/1
  Gain3/1 -> Product5/1
  Gain2/1 -> Product6/1
  Demux3/2 -> Sum1/2
  Gain1/1 -> Product3/1
  Sum1/1 -> Gain1/1
  Sum/1 -> "[3*1]"/1
  Product3/1 -> Sum/1
  Product5/1 -> Sum/3
  Product6/1 -> Sum/2
  "[0;0;1]"/1 -> Product5/2
  "[0;1;0]"/1 -> Product6/2
  "[1;0;0]"/1 -> Product3/2
  Demux3/1 -> Sum2/2
  Demux3/3 -> Terminator3/1
  Product2/1 -> Demux3/1
  "[0;0;1]1"/1 -> Product2/2
  Demux2/1 -> Terminator1/1
  Product1/1 -> Demux2/1
  "[1;0;0]1"/1 -> Product1/2
  Demux1/3 -> Sum1/1
  Demux1/2 -> Terminator2/1
  Product4/1 -> Demux1/1
  "[0;1;0]1"/1 -> Product4/2
  "[3*3]"/1 -> Product1/1, Product2/1, Product4/1

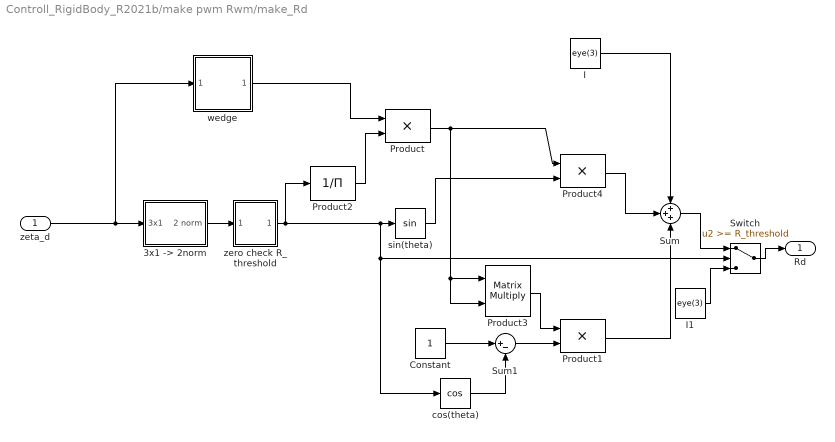
== system Controll_RigidBody_R2021b/make pwm Rwm/make_Rd ==
  zeta_d : Inport
  "3x1 -> 2norm" : Subsystem
  Constant : Constant
  I : Constant  Value=eye(3)  VectorParams1D=off
  I1 : Constant  Value=eye(3)  VectorParams1D=off
  Product : Product  InputSameDT=on  SaturateOnIntegerOverflow=on  OutDataTypeStr=Inherit: Same as first input
  Product1 : Product  InputSameDT=on  SaturateOnIntegerOverflow=on  OutDataTypeStr=Inherit: Same as first input
  Product2 : Product  Inputs=/  InputSameDT=on  SaturateOnIntegerOverflow=on  OutDataTypeStr=Inherit: Same as first input
  Product3 : Product  Multiplication=Matrix(*)  InputSameDT=on  SaturateOnIntegerOverflow=on  OutDataTypeStr=Inherit: Same as first input
  Product4 : Product  InputSameDT=on  SaturateOnIntegerOverflow=on  OutDataTypeStr=Inherit: Same as first input
  Sum : Sum  Inputs=+++  InputSameDT=on  SaturateOnIntegerOverflow=on  OutDataTypeStr=Inherit: Same as first input
  Sum1 : Sum  Inputs=|+-  InputSameDT=on  SaturateOnIntegerOverflow=on  OutDataTypeStr=Inherit: Same as first input
  Switch : Switch  Threshold=R_threshold  SaturateOnIntegerOverflow=on  InputSameDT=on
  cos(theta) : Trigonometry  Operator=cos
  sin(theta) : Trigonometry
  wedge : Subsystem
  zero check R_threshold : Subsystem
  Rd : Outport  VectorParamsAs1DForOutWhenUnconnected=off
  wires:
  Product3/1 -> Product1/1
  zeta_d/1 -> wedge/1("[3x1]"), "3x1 -> 2norm"/1(3x1)
  Product2/1 -> Product/2
  zero check R_threshold/1(Out1) -> cos(theta)/1, Switch/2, sin(theta)/1, Product2/1
  wedge/1("[3x3]") -> Product/1
  Product/1 -> Product3/2, Product3/1, Product4/1
  "3x1 -> 2norm"/1(2 norm) -> zero check R_threshold/1(In1)
  Switch/1 -> Rd/1
  I1/1 -> Switch/3
  Sum/1 -> Switch/1
  sin(theta)/1 -> Product4/2
  I/1 -> Sum/1
  Constant/1 -> Sum1/1
  cos(theta)/1 -> Sum1/2
  Sum1/1 -> Product1/2
  Product1/1 -> Sum/3
  Product4/1 -> Sum/2

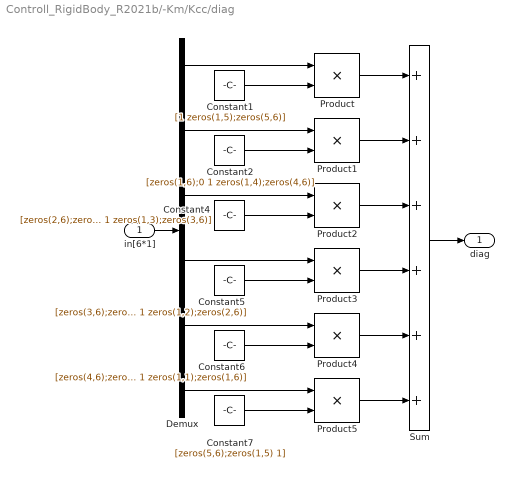
== system Controll_RigidBody_R2021b/-Km/Kcc/diag ==
  in[6*1] : Inport
  Constant1 : Constant  Value=[1 zeros(1,5);zeros(5,6)]  VectorParams1D=off
  Constant2 : Constant  Value=[zeros(1,6);0 1 zeros(1,4);zeros(4,6)]  VectorParams1D=off
  Constant4 : Constant  Value=[zeros(2,6);zeros(1,2) 1 zeros(1,3);zeros(3,6)]  VectorParams1D=off
  Constant5 : Constant  Value=[zeros(3,6);zeros(1,3) 1 zeros(1,2);zeros(2,6)]  VectorParams1D=off
  Constant6 : Constant  Value=[zeros(4,6);zeros(1,4) 1 zeros(1,1);zeros(1,6)]  VectorParams1D=off
  Constant7 : Constant  Value=[zeros(5,6);zeros(1,5) 1]  VectorParams1D=off
  Demux : Demux  Outputs=6
      settings: DisplayOption=none
  Product{,1..5} (6 alike) : Product  InputSameDT=on  SaturateOnIntegerOverflow=on  OutDataTypeStr=Inherit: Same as first input
  Sum : Sum  Inputs=++++++  InputSameDT=on  SaturateOnIntegerOverflow=on  OutDataTypeStr=Inherit: Same as first input
  diag : Outport  VectorParamsAs1DForOutWhenUnconnected=off
  wires:
  Demux/1 -> Product/1
  Constant1/1 -> Product/2
  Demux/2 -> Product1/1
  Constant2/1 -> Product1/2
  Demux/3 -> Product2/1
  Constant4/1 -> Product2/2
  Demux/4 -> Product3/1
  Constant5/1 -> Product3/2
  Constant6/1 -> Product4/2
  Demux/5 -> Product4/1
  Constant7/1 -> Product5/2
  Demux/6 -> Product5/1
  Product5/1 -> Sum/6
  Product4/1 -> Sum/5
  Product3/1 -> Sum/4
  Product2/1 -> Sum/3
  Product1/1 -> Sum/2
  Product/1 -> Sum/1
  in[6*1]/1 -> Demux/1
  Sum/1 -> diag/1

== system Controll_RigidBody_R2021b/Rd to zetad/e_R(R)/sk(R) ==
  R : Inport
  Gain : Gain  Gain=1/2  SaturateOnIntegerOverflow=on  OutDataTypeStr=Inherit: Same as input  ParamDataTypeStr=Inherit: Same as input
  Math Function2 : Math  Operator=transpose  SignedPower=on  SaturateOnIntegerOverflow=on
  Sum : Sum  Inputs=|+-  InputSameDT=on  SaturateOnIntegerOverflow=on  OutDataTypeStr=Inherit: Same as first input
  sk(R) : Outport  VectorParamsAs1DForOutWhenUnconnected=off
  wires:
  Gain/1 -> sk(R)/1
  Sum/1 -> Gain/1
  Math Function2/1 -> Sum/2
  R/1 -> Sum/1, Math Function2/1

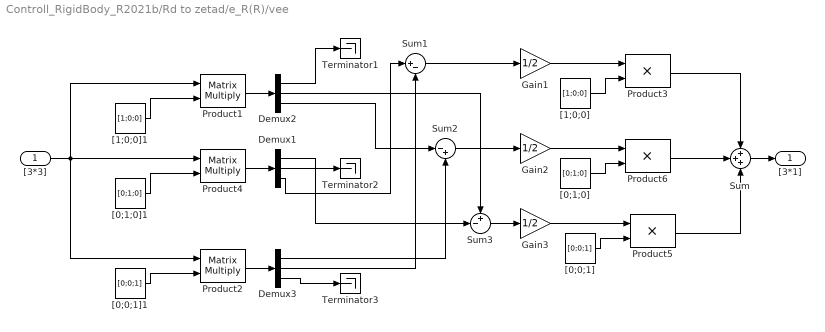
== system Controll_RigidBody_R2021b/Rd to zetad/e_R(R)/vee ==
  "[3*3]" : Inport
  Demux1 : Demux  Outputs=3
      settings: DisplayOption=none
  Demux2 : Demux  Outputs=3
      settings: DisplayOption=none
  Demux3 : Demux  Outputs=3
      settings: DisplayOption=none
  Gain1 : Gain  Gain=1/2  SaturateOnIntegerOverflow=on  OutDataTypeStr=Inherit: Same as input  ParamDataTypeStr=Inherit: Same as input
  Gain2 : Gain  Gain=1/2  SaturateOnIntegerOverflow=on  OutDataTypeStr=Inherit: Same as input  ParamDataTypeStr=Inherit: Same as input
  Gain3 : Gain  Gain=1/2  SaturateOnIntegerOverflow=on  OutDataTypeStr=Inherit: Same as input  ParamDataTypeStr=Inherit: Same as input
  Product1 : Product  Multiplication=Matrix(*)  InputSameDT=on  SaturateOnIntegerOverflow=on  OutDataTypeStr=Inherit: Same as first input
  Product2 : Product  Multiplication=Matrix(*)  InputSameDT=on  SaturateOnIntegerOverflow=on  OutDataTypeStr=Inherit: Same as first input
  Product3 : Product  InputSameDT=on  SaturateOnIntegerOverflow=on  OutDataTypeStr=Inherit: Same as first input
  Product4 : Product  Multiplication=Matrix(*)  InputSameDT=on  SaturateOnIntegerOverflow=on  OutDataTypeStr=Inherit: Same as first input
  Product5 : Product  InputSameDT=on  SaturateOnIntegerOverflow=on  OutDataTypeStr=Inherit: Same as first input
  Product6 : Product  InputSameDT=on  SaturateOnIntegerOverflow=on  OutDataTypeStr=Inherit: Same as first input
  Sum : Sum  Inputs=+++  InputSameDT=on  SaturateOnIntegerOverflow=on  OutDataTypeStr=Inherit: Same as first input
  Sum1 : Sum  Inputs=|+-  InputSameDT=on  SaturateOnIntegerOverflow=on  OutDataTypeStr=Inherit: Same as first input
  Sum2 : Sum  Inputs=|-+  InputSameDT=on  SaturateOnIntegerOverflow=on  OutDataTypeStr=Inherit: Same as first input
  Sum3 : Sum  Inputs=+-|  InputSameDT=on  SaturateOnIntegerOverflow=on  OutDataTypeStr=Inherit: Same as first input
  Terminator1 : Terminator
  Terminator2 : Terminator
  Terminator3 : Terminator
  "[0;0;1]" : Constant  Value=[0;0;1]  VectorParams1D=off
  "[0;0;1]1" : Constant  Value=[0;0;1]  VectorParams1D=off
  "[0;1;0]" : Constant  Value=[0;1;0]  VectorParams1D=off
  "[0;1;0]1" : Constant  Value=[0;1;0]  VectorParams1D=off
  "[1;0;0]" : Constant  Value=[1;0;0]  VectorParams1D=off
  "[1;0;0]1" : Constant  Value=[1;0;0]  VectorParams1D=off
  "[3*1]" : Outport  VectorParamsAs1DForOutWhenUnconnected=off
  wires:
  Demux1/1 -> Sum3/2
  Demux2/2 -> Sum3/1
  Sum3/1 -> Gain3/1
  Sum2/1 -> Gain2/1
  Demux2/3 -> Sum2/1
  Gain3/1 -> Product5/1
  Gain2/1 -> Product6/1
  Demux3/2 -> Sum1/2
  Gain1/1 -> Product3/1
  Sum1/1 -> Gain1/1
  Sum/1 -> "[3*1]"/1
  Product3/1 -> Sum/1
  Product5/1 -> Sum/3
  Product6/1 -> Sum/2
  "[0;0;1]"/1 -> Product5/2
  "[0;1;0]"/1 -> Product6/2
  "[1;0;0]"/1 -> Product3/2
  Demux3/1 -> Sum2/2
  Demux3/3 -> Terminator3/1
  Product2/1 -> Demux3/1
  "[0;0;1]1"/1 -> Product2/2
  Demux2/1 -> Terminator1/1
  Product1/1 -> Demux2/1
  "[1;0;0]1"/1 -> Product1/2
  Demux1/3 -> Sum1/1
  Demux1/2 -> Terminator2/1
  Product4/1 -> Demux1/1
  "[0;1;0]1"/1 -> Product4/2
  "[3*3]"/1 -> Product1/1, Product2/1, Product4/1

== system Controll_RigidBody_R2021b/Rd to zetad/make zeta/3x1 -> 2norm ==
  3x1 : Inport
  Demux : Demux  Outputs=3
      settings: DisplayOption=none
  Math Function : Math  Operator=magnitude^2  SignedPower=on  SaturateOnIntegerOverflow=on
  Math Function1 : Math  Operator=sqrt  SignedPower=on  SaturateOnIntegerOverflow=on
  Sum : Sum  Inputs=+++  InputSameDT=on  SaturateOnIntegerOverflow=on  OutDataTypeStr=Inherit: Same as first input
  2 norm : Outport  VectorParamsAs1DForOutWhenUnconnected=off
  wires:
  3x1/1 -> Math Function/1
  Math Function1/1 -> 2 norm/1
  Sum/1 -> Math Function1/1
  Demux/1 -> Sum/1
  Demux/2 -> Sum/2
  Demux/3 -> Sum/3
  Math Function/1 -> Demux/1

== system Controll_RigidBody_R2021b/Rd to zetad/make zeta/zero check zeta_threshold ==
  In1 : Inport
  Switch : Switch  Threshold=zeta_threshold  SaturateOnIntegerOverflow=on  InputSameDT=on
  norm_eR : Constant  Value=zeta_threshold  VectorParams1D=off
  Out1 : Outport  VectorParamsAs1DForOutWhenUnconnected=off
  wires:
  Switch/1 -> Out1/1
  In1/1 -> Switch/2, Switch/1
  norm_eR/1 -> Switch/3

== system Controll_RigidBody_R2021b/Rwm to zetawm/e_R(R)/sk(R) ==
  R : Inport
  Gain : Gain  Gain=1/2  SaturateOnIntegerOverflow=on  OutDataTypeStr=Inherit: Same as input  ParamDataTypeStr=Inherit: Same as input
  Math Function2 : Math  Operator=transpose  SignedPower=on  SaturateOnIntegerOverflow=on
  Sum : Sum  Inputs=|+-  InputSameDT=on  SaturateOnIntegerOverflow=on  OutDataTypeStr=Inherit: Same as first input
  sk(R) : Outport  VectorParamsAs1DForOutWhenUnconnected=off
  wires:
  Gain/1 -> sk(R)/1
  Sum/1 -> Gain/1
  Math Function2/1 -> Sum/2
  R/1 -> Sum/1, Math Function2/1

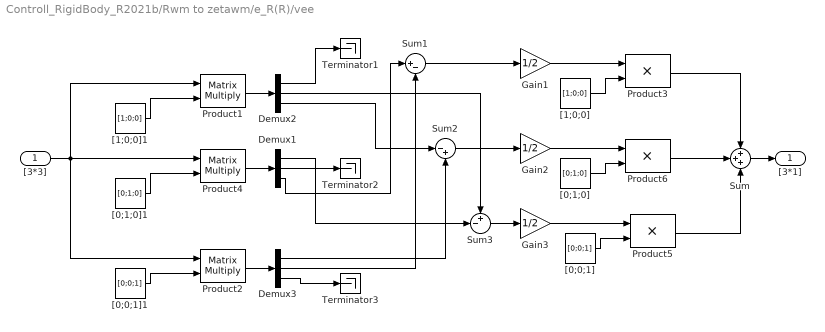
== system Controll_RigidBody_R2021b/Rwm to zetawm/e_R(R)/vee ==
  "[3*3]" : Inport
  Demux1 : Demux  Outputs=3
      settings: DisplayOption=none
  Demux2 : Demux  Outputs=3
      settings: DisplayOption=none
  Demux3 : Demux  Outputs=3
      settings: DisplayOption=none
  Gain1 : Gain  Gain=1/2  SaturateOnIntegerOverflow=on  OutDataTypeStr=Inherit: Same as input  ParamDataTypeStr=Inherit: Same as input
  Gain2 : Gain  Gain=1/2  SaturateOnIntegerOverflow=on  OutDataTypeStr=Inherit: Same as input  ParamDataTypeStr=Inherit: Same as input
  Gain3 : Gain  Gain=1/2  SaturateOnIntegerOverflow=on  OutDataTypeStr=Inherit: Same as input  ParamDataTypeStr=Inherit: Same as input
  Product1 : Product  Multiplication=Matrix(*)  InputSameDT=on  SaturateOnIntegerOverflow=on  OutDataTypeStr=Inherit: Same as first input
  Product2 : Product  Multiplication=Matrix(*)  InputSameDT=on  SaturateOnIntegerOverflow=on  OutDataTypeStr=Inherit: Same as first input
  Product3 : Product  InputSameDT=on  SaturateOnIntegerOverflow=on  OutDataTypeStr=Inherit: Same as first input
  Product4 : Product  Multiplication=Matrix(*)  InputSameDT=on  SaturateOnIntegerOverflow=on  OutDataTypeStr=Inherit: Same as first input
  Product5 : Product  InputSameDT=on  SaturateOnIntegerOverflow=on  OutDataTypeStr=Inherit: Same as first input
  Product6 : Product  InputSameDT=on  SaturateOnIntegerOverflow=on  OutDataTypeStr=Inherit: Same as first input
  Sum : Sum  Inputs=+++  InputSameDT=on  SaturateOnIntegerOverflow=on  OutDataTypeStr=Inherit: Same as first input
  Sum1 : Sum  Inputs=|+-  InputSameDT=on  SaturateOnIntegerOverflow=on  OutDataTypeStr=Inherit: Same as first input
  Sum2 : Sum  Inputs=|-+  InputSameDT=on  SaturateOnIntegerOverflow=on  OutDataTypeStr=Inherit: Same as first input
  Sum3 : Sum  Inputs=+-|  InputSameDT=on  SaturateOnIntegerOverflow=on  OutDataTypeStr=Inherit: Same as first input
  Terminator1 : Terminator
  Terminator2 : Terminator
  Terminator3 : Terminator
  "[0;0;1]" : Constant  Value=[0;0;1]  VectorParams1D=off
  "[0;0;1]1" : Constant  Value=[0;0;1]  VectorParams1D=off
  "[0;1;0]" : Constant  Value=[0;1;0]  VectorParams1D=off
  "[0;1;0]1" : Constant  Value=[0;1;0]  VectorParams1D=off
  "[1;0;0]" : Constant  Value=[1;0;0]  VectorParams1D=off
  "[1;0;0]1" : Constant  Value=[1;0;0]  VectorParams1D=off
  "[3*1]" : Outport  VectorParamsAs1DForOutWhenUnconnected=off
  wires:
  Demux1/1 -> Sum3/2
  Demux2/2 -> Sum3/1
  Sum3/1 -> Gain3/1
  Sum2/1 -> Gain2/1
  Demux2/3 -> Sum2/1
  Gain3/1 -> Product5/1
  Gain2/1 -> Product6/1
  Demux3/2 -> Sum1/2
  Gain1/1 -> Product3/1
  Sum1/1 -> Gain1/1
  Sum/1 -> "[3*1]"/1
  Product3/1 -> Sum/1
  Product5/1 -> Sum/3
  Product6/1 -> Sum/2
  "[0;0;1]"/1 -> Product5/2
  "[0;1;0]"/1 -> Product6/2
  "[1;0;0]"/1 -> Product3/2
  Demux3/1 -> Sum2/2
  Demux3/3 -> Terminator3/1
  Product2/1 -> Demux3/1
  "[0;0;1]1"/1 -> Product2/2
  Demux2/1 -> Terminator1/1
  Product1/1 -> Demux2/1
  "[1;0;0]1"/1 -> Product1/2
  Demux1/3 -> Sum1/1
  Demux1/2 -> Terminator2/1
  Product4/1 -> Demux1/1
  "[0;1;0]1"/1 -> Product4/2
  "[3*3]"/1 -> Product1/1, Product2/1, Product4/1

== system Controll_RigidBody_R2021b/Rwm to zetawm/make zeta/3x1 -> 2norm ==
  3x1 : Inport
  Demux : Demux  Outputs=3
      settings: DisplayOption=none
  Math Function : Math  Operator=magnitude^2  SignedPower=on  SaturateOnIntegerOverflow=on
  Math Function1 : Math  Operator=sqrt  SignedPower=on  SaturateOnIntegerOverflow=on
  Sum : Sum  Inputs=+++  InputSameDT=on  SaturateOnIntegerOverflow=on  OutDataTypeStr=Inherit: Same as first input
  2 norm : Outport  VectorParamsAs1DForOutWhenUnconnected=off
  wires:
  3x1/1 -> Math Function/1
  Math Function1/1 -> 2 norm/1
  Sum/1 -> Math Function1/1
  Demux/1 -> Sum/1
  Demux/2 -> Sum/2
  Demux/3 -> Sum/3
  Math Function/1 -> Demux/1

== system Controll_RigidBody_R2021b/Rwm to zetawm/make zeta/zero check zeta_threshold ==
  In1 : Inport
  Switch : Switch  Threshold=zeta_threshold  SaturateOnIntegerOverflow=on  InputSameDT=on
  norm_eR : Constant  Value=zeta_threshold  VectorParams1D=off
  Out1 : Outport  VectorParamsAs1DForOutWhenUnconnected=off
  wires:
  Switch/1 -> Out1/1
  In1/1 -> Switch/2, Switch/1
  norm_eR/1 -> Switch/3

== system Controll_RigidBody_R2021b/Rwm to zetawm1/e_R(R)/sk(R) ==
  R : Inport
  Gain : Gain  Gain=1/2  SaturateOnIntegerOverflow=on  OutDataTypeStr=Inherit: Same as input  ParamDataTypeStr=Inherit: Same as input
  Math Function2 : Math  Operator=transpose  SignedPower=on  SaturateOnIntegerOverflow=on
  Sum : Sum  Inputs=|+-  InputSameDT=on  SaturateOnIntegerOverflow=on  OutDataTypeStr=Inherit: Same as first input
  sk(R) : Outport  VectorParamsAs1DForOutWhenUnconnected=off
  wires:
  Gain/1 -> sk(R)/1
  Sum/1 -> Gain/1
  Math Function2/1 -> Sum/2
  R/1 -> Sum/1, Math Function2/1

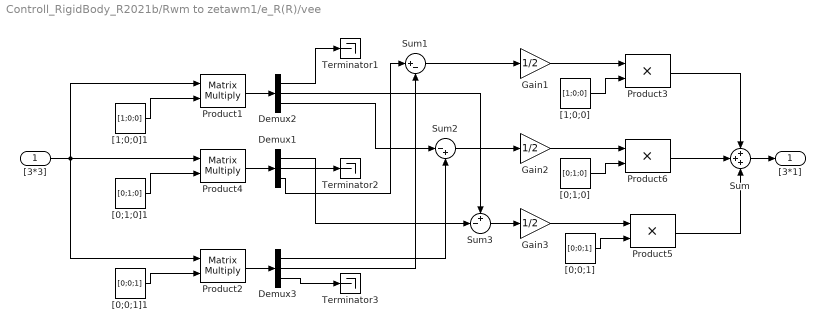
== system Controll_RigidBody_R2021b/Rwm to zetawm1/e_R(R)/vee ==
  "[3*3]" : Inport
  Demux1 : Demux  Outputs=3
      settings: DisplayOption=none
  Demux2 : Demux  Outputs=3
      settings: DisplayOption=none
  Demux3 : Demux  Outputs=3
      settings: DisplayOption=none
  Gain1 : Gain  Gain=1/2  SaturateOnIntegerOverflow=on  OutDataTypeStr=Inherit: Same as input  ParamDataTypeStr=Inherit: Same as input
  Gain2 : Gain  Gain=1/2  SaturateOnIntegerOverflow=on  OutDataTypeStr=Inherit: Same as input  ParamDataTypeStr=Inherit: Same as input
  Gain3 : Gain  Gain=1/2  SaturateOnIntegerOverflow=on  OutDataTypeStr=Inherit: Same as input  ParamDataTypeStr=Inherit: Same as input
  Product1 : Product  Multiplication=Matrix(*)  InputSameDT=on  SaturateOnIntegerOverflow=on  OutDataTypeStr=Inherit: Same as first input
  Product2 : Product  Multiplication=Matrix(*)  InputSameDT=on  SaturateOnIntegerOverflow=on  OutDataTypeStr=Inherit: Same as first input
  Product3 : Product  InputSameDT=on  SaturateOnIntegerOverflow=on  OutDataTypeStr=Inherit: Same as first input
  Product4 : Product  Multiplication=Matrix(*)  InputSameDT=on  SaturateOnIntegerOverflow=on  OutDataTypeStr=Inherit: Same as first input
  Product5 : Product  InputSameDT=on  SaturateOnIntegerOverflow=on  OutDataTypeStr=Inherit: Same as first input
  Product6 : Product  InputSameDT=on  SaturateOnIntegerOverflow=on  OutDataTypeStr=Inherit: Same as first input
  Sum : Sum  Inputs=+++  InputSameDT=on  SaturateOnIntegerOverflow=on  OutDataTypeStr=Inherit: Same as first input
  Sum1 : Sum  Inputs=|+-  InputSameDT=on  SaturateOnIntegerOverflow=on  OutDataTypeStr=Inherit: Same as first input
  Sum2 : Sum  Inputs=|-+  InputSameDT=on  SaturateOnIntegerOverflow=on  OutDataTypeStr=Inherit: Same as first input
  Sum3 : Sum  Inputs=+-|  InputSameDT=on  SaturateOnIntegerOverflow=on  OutDataTypeStr=Inherit: Same as first input
  Terminator1 : Terminator
  Terminator2 : Terminator
  Terminator3 : Terminator
  "[0;0;1]" : Constant  Value=[0;0;1]  VectorParams1D=off
  "[0;0;1]1" : Constant  Value=[0;0;1]  VectorParams1D=off
  "[0;1;0]" : Constant  Value=[0;1;0]  VectorParams1D=off
  "[0;1;0]1" : Constant  Value=[0;1;0]  VectorParams1D=off
  "[1;0;0]" : Constant  Value=[1;0;0]  VectorParams1D=off
  "[1;0;0]1" : Constant  Value=[1;0;0]  VectorParams1D=off
  "[3*1]" : Outport  VectorParamsAs1DForOutWhenUnconnected=off
  wires:
  Demux1/1 -> Sum3/2
  Demux2/2 -> Sum3/1
  Sum3/1 -> Gain3/1
  Sum2/1 -> Gain2/1
  Demux2/3 -> Sum2/1
  Gain3/1 -> Product5/1
  Gain2/1 -> Product6/1
  Demux3/2 -> Sum1/2
  Gain1/1 -> Product3/1
  Sum1/1 -> Gain1/1
  Sum/1 -> "[3*1]"/1
  Product3/1 -> Sum/1
  Product5/1 -> Sum/3
  Product6/1 -> Sum/2
  "[0;0;1]"/1 -> Product5/2
  "[0;1;0]"/1 -> Product6/2
  "[1;0;0]"/1 -> Product3/2
  Demux3/1 -> Sum2/2
  Demux3/3 -> Terminator3/1
  Product2/1 -> Demux3/1
  "[0;0;1]1"/1 -> Product2/2
  Demux2/1 -> Terminator1/1
  Product1/1 -> Demux2/1
  "[1;0;0]1"/1 -> Product1/2
  Demux1/3 -> Sum1/1
  Demux1/2 -> Terminator2/1
  Product4/1 -> Demux1/1
  "[0;1;0]1"/1 -> Product4/2
  "[3*3]"/1 -> Product1/1, Product2/1, Product4/1

== system Controll_RigidBody_R2021b/Rwm to zetawm1/make zeta/3x1 -> 2norm ==
  3x1 : Inport
  Demux : Demux  Outputs=3
      settings: DisplayOption=none
  Math Function : Math  Operator=magnitude^2  SignedPower=on  SaturateOnIntegerOverflow=on
  Math Function1 : Math  Operator=sqrt  SignedPower=on  SaturateOnIntegerOverflow=on
  Sum : Sum  Inputs=+++  InputSameDT=on  SaturateOnIntegerOverflow=on  OutDataTypeStr=Inherit: Same as first input
  2 norm : Outport  VectorParamsAs1DForOutWhenUnconnected=off
  wires:
  3x1/1 -> Math Function/1
  Math Function1/1 -> 2 norm/1
  Sum/1 -> Math Function1/1
  Demux/1 -> Sum/1
  Demux/2 -> Sum/2
  Demux/3 -> Sum/3
  Math Function/1 -> Demux/1

== system Controll_RigidBody_R2021b/Rwm to zetawm1/make zeta/zero check zeta_threshold ==
  In1 : Inport
  Switch : Switch  Threshold=zeta_threshold  SaturateOnIntegerOverflow=on  InputSameDT=on
  norm_eR : Constant  Value=zeta_threshold  VectorParams1D=off
  Out1 : Outport  VectorParamsAs1DForOutWhenUnconnected=off
  wires:
  Switch/1 -> Out1/1
  In1/1 -> Switch/2, Switch/1
  norm_eR/1 -> Switch/3

== system Controll_RigidBody_R2021b/make Rd pd/make_Rd/3x1 -> 2norm ==
  3x1 : Inport
  Demux : Demux  Outputs=3
      settings: DisplayOption=none
  Math Function : Math  Operator=magnitude^2  SignedPower=on  SaturateOnIntegerOverflow=on
  Math Function1 : Math  Operator=sqrt  SignedPower=on  SaturateOnIntegerOverflow=on
  Sum : Sum  Inputs=+++  InputSameDT=on  SaturateOnIntegerOverflow=on  OutDataTypeStr=Inherit: Same as first input
  2 norm : Outport  VectorParamsAs1DForOutWhenUnconnected=off
  wires:
  Math Function/1 -> Demux/1
  Demux/3 -> Sum/3
  Demux/2 -> Sum/2
  Demux/1 -> Sum/1
  Sum/1 -> Math Function1/1
  Math Function1/1 -> 2 norm/1
  3x1/1 -> Math Function/1

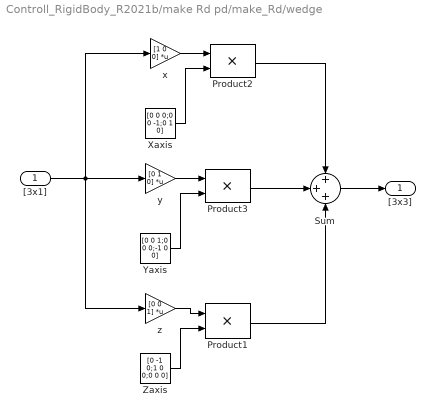
== system Controll_RigidBody_R2021b/make Rd pd/make_Rd/wedge ==
  "[3x1]" : Inport
  Product1 : Product  InputSameDT=on  SaturateOnIntegerOverflow=on  OutDataTypeStr=Inherit: Same as first input
  Product2 : Product  InputSameDT=on  SaturateOnIntegerOverflow=on  OutDataTypeStr=Inherit: Same as first input
  Product3 : Product  InputSameDT=on  SaturateOnIntegerOverflow=on  OutDataTypeStr=Inherit: Same as first input
  Sum : Sum  Inputs=+++  InputSameDT=on  SaturateOnIntegerOverflow=on  OutDataTypeStr=Inherit: Same as first input
  Xaxis : Constant  Value=[0 0 0;0 0 -1;0 1 0]  VectorParams1D=off
  Yaxis : Constant  Value=[0 0 1;0 0 0;-1 0 0]  VectorParams1D=off
  Zaxis : Constant  Value=[0 -1 0;1 0 0;0 0 0]  VectorParams1D=off
  x : Gain  Gain=[1 0 0]  Multiplication=Matrix(K*u)  SaturateOnIntegerOverflow=on  OutDataTypeStr=Inherit: Same as input  ParamDataTypeStr=Inherit: Same as input
  y : Gain  Gain=[0 1 0]  Multiplication=Matrix(K*u)  SaturateOnIntegerOverflow=on  OutDataTypeStr=Inherit: Same as input  ParamDataTypeStr=Inherit: Same as input
  z : Gain  Gain=[0 0 1]  Multiplication=Matrix(K*u)  SaturateOnIntegerOverflow=on  OutDataTypeStr=Inherit: Same as input  ParamDataTypeStr=Inherit: Same as input
  "[3x3]" : Outport  VectorParamsAs1DForOutWhenUnconnected=off
  wires:
  Sum/1 -> "[3x3]"/1
  Product1/1 -> Sum/3
  Product2/1 -> Sum/1
  Product3/1 -> Sum/2
  "[3x1]"/1 -> z/1, x/1, y/1
  y/1 -> Product3/1
  Yaxis/1 -> Product3/2
  x/1 -> Product2/1
  Xaxis/1 -> Product2/2
  z/1 -> Product1/1
  Zaxis/1 -> Product1/2

== system Controll_RigidBody_R2021b/make Rd pd/make_Rd/zero check R_threshold ==
  In1 : Inport
  Switch : Switch  Threshold=R_threshold  SaturateOnIntegerOverflow=on  InputSameDT=on
  norm_xi : Constant  Value=R_threshold  VectorParams1D=off
  Out1 : Outport  VectorParamsAs1DForOutWhenUnconnected=off
  wires:
  Switch/1 -> Out1/1
  In1/1 -> Switch/2, Switch/1
  norm_xi/1 -> Switch/3
